simulink model "prova02"  (R2022b)
settings: Solver=VariableStepAuto  StartTime=0.0  StopTime=20  RelTol=1e-3
settings Model: Creator=giaco  LastModifiedBy=giaco

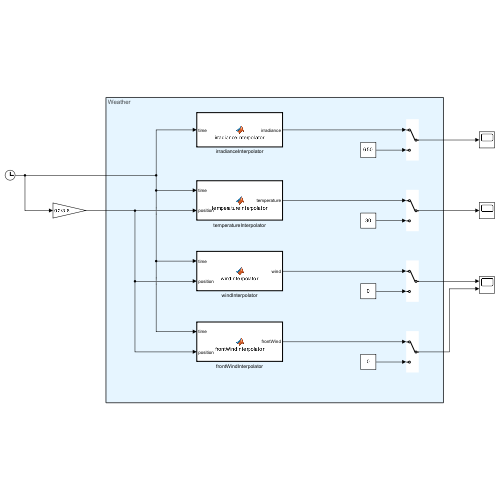
[thumbnail: Simulink's stored preview of the top-level diagram]
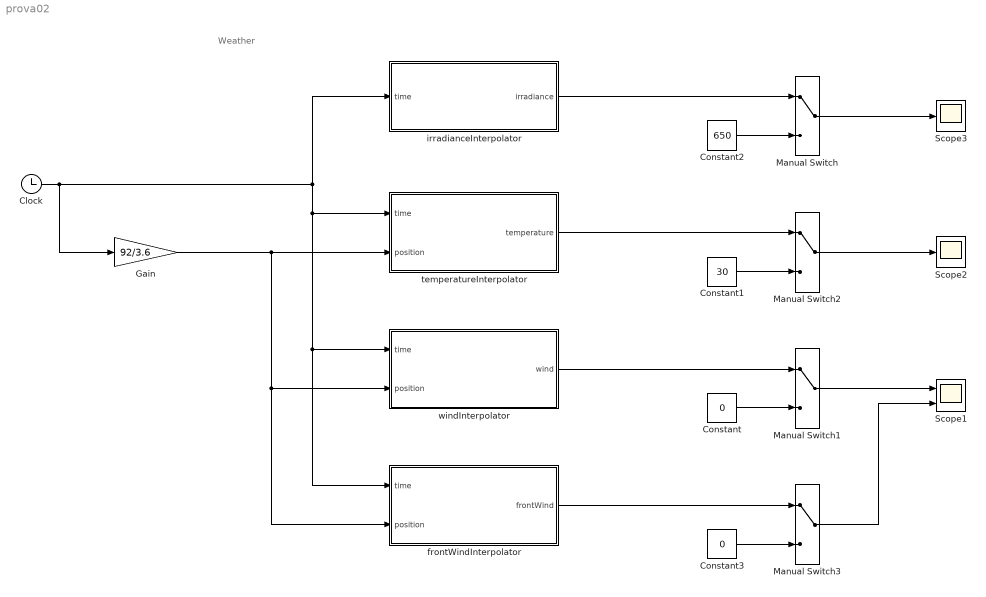
== system prova02 ==
  note: Weather
  Clock : Clock
  Constant : Constant  Value=0
  Constant1 : Constant  Value=30
  Constant2 : Constant  Value=650
  Constant3 : Constant  Value=0
  Gain : Gain  Gain=92/3.6
  Manual Switch{,1..3} (4 alike) : ManualSwitch
  Scope1 : Scope  NumInputPorts=2
  Scope2 : Scope
  Scope3 : Scope
  frontWindInterpolator : MATLAB Function  TreatAsAtomicUnit=on
  irradianceInterpolator : MATLAB Function  TreatAsAtomicUnit=on
  temperatureInterpolator : MATLAB Function  TreatAsAtomicUnit=on
  windInterpolator : MATLAB Function  TreatAsAtomicUnit=on
  wires:
  Constant2/1 -> Manual Switch/2
  Constant3/1 -> Manual Switch3/2
  Constant/1 -> Manual Switch1/2
  temperatureInterpolator/1(temperature) -> Manual Switch2/1
  windInterpolator/1(wind) -> Manual Switch1/1
  Constant1/1 -> Manual Switch2/2
  frontWindInterpolator/1(frontWind) -> Manual Switch3/1
  irradianceInterpolator/1(irradiance) -> Manual Switch/1
  Manual Switch2/1 -> Scope2/1
  Manual Switch1/1 -> Scope1/1
  Manual Switch3/1 -> Scope1/2
  Manual Switch/1 -> Scope3/1
  Gain/1 -> frontWindInterpolator/2(position), windInterpolator/2(position), temperatureInterpolator/2(position)
  Clock/1 -> irradianceInterpolator/1(time), frontWindInterpolator/1(time), windInterpolator/1(time), temperatureInterpolator/1(time), Gain/1

== matlab function prova02/temperatureInterpolator ==
  data: time input; position input; temperature output; weatherSim parameter
function temperature = temperatureInterpolator(time, position, weatherSim)

coder.extrinsic('temperatureInterpolant');

temperature = nan(1, 1);

temperature(1) = temperatureInterpolant(time, position, weatherSim);

== matlab function prova02/irradianceInterpolator ==
  data: time input; irradiance output; weatherSim parameter
function irradiance = irradianceInterpolator(time, weatherSim)

coder.extrinsic('irradianceInterpolant');

irradiance = nan(1, 1);

irradiance(1) = irradianceInterpolant(time, weatherSim);

== matlab function prova02/frontWindInterpolator ==
  data: time input; position input; frontWind output; weatherSim parameter
function frontWind = frontWindInterpolator(time, position, weatherSim)

coder.extrinsic('frontWindInterpolant');

frontWind = nan(1, 1);

frontWind(1) = frontWindInterpolant(time, position, weatherSim);

== matlab function prova02/windInterpolator ==
  data: time input; position input; wind output; weatherSim parameter
function wind = windInterpolator(time, position, weatherSim)

coder.extrinsic('windInterpolant');

wind = nan(1, 1);

wind(1) = windInterpolant(time, position, weatherSim);
